simulink model "Aircraft_Power_Network"  (R2015a)
settings: Solver=ode23t  StartTime=0.0  StopTime=40  RelTol=1e-3
PostLoadFcn:
  | %load PQ_DATA4
  | Flight_Cycle_Num = 1;
  | 
  | warning off Simulink:blocks:MatchingFromNotFound
  | warning off Simulink:blocks:MatchingGotoNotFound
  | warning off Simulink:Engine:SaveWithParameterizedLinks_Warning
  | warning off MATLAB:nearlySingularMatrix
  | warning off simscape:compiler:sli:init:SolverNotRecommended
  | warning off Simulink:ID:DuplicateSID
  | warning off Simulink:Engine:UINotUpdatedDuringRapidAccelSim
  | warning off Simulink:SampleTime:IllegalIPortRateTrans
  | warning off Simulink:SampleTime:SourceInheritedTS
StartFcn:
  | tic;
StopFcn:
  | Elapsed_Sim_Time = toc; disp(['Elapsed time is ' num2str(Elapsed_Sim_Time)])
undefined symbols (not defined in the file): sigbuilder_block, Ts
libraries: powerlib x6, powerlib_meascontrol x4, Actuator_AC_Lib x2, Lamp_Lib x2, Pump_Lib x2, DC_Loads_Lib x2, Distribution_Lib x1, Generator_Lib x1, Power_Calc_Lib x1
Description:
  | Copyright 2014 The MathWorks, Inc.
settings Model: CovSFcnEnable=off  TunableVars=Flight_Cycle_Num  TunableVarsStorageClass=Auto  Creator=smiller  LastModifiedBy=dmeissne
settings OptimizationCC: InlineParams=on  OptimizeBlockIOStorage=off  BufferReuse=off  GlobalBufferReuse=off  ExpressionFolding=off  LocalBlockOutputs=off
settings DebuggingCC: UnderspecifiedInitializationDetection=Classic  MergeDetectMultiDrivingBlocksExec=none  SolverPrmCheckMsg=warning  MultiTaskRateTransMsg=warning  StateNameClashWarn=warning
settings GRTTargetCC: CombineOutputUpdateFcns=off  GRTInterface=on

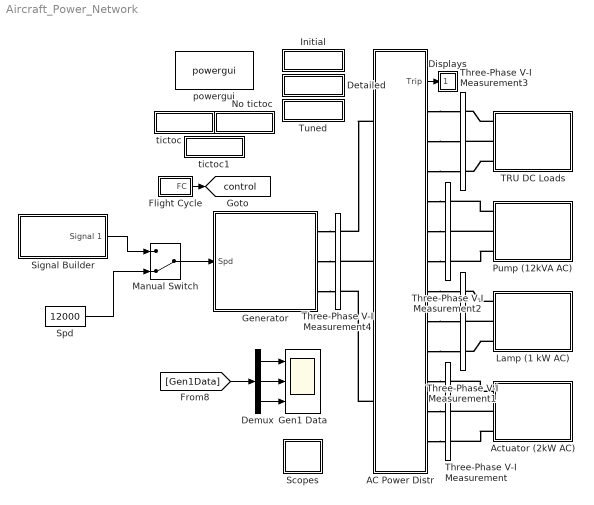
== system Aircraft_Power_Network ==
  AC Power Distr : Subsystem  BlockChoice=Phasor
      settings: AttributesFormatString=%<BlockChoice>  TemplateBlock=Distribution_Lib/AC Power Distr  MemberBlocks=Detailed,Phasor
  Actuator (2kW AC) : Subsystem  BlockChoice=Phasor
      link override Detailed/PM Synchronous Motor Drive/Output Bus Selector: OutputSignals=Rotor speed wm (rad/s)
      link override Detailed/PM Synchronous Motor Drive/Permanent Magnet Synchronous Machine: MechanicalLoad=Torque Tm  VoltageCst=126.966  TorqueCst=1.05
      link override Phasor/Calc PQ: BlockChoice=Tuned
      settings: AttributesFormatString=%<BlockChoice>  TemplateBlock=Actuator_AC_Lib/Actuator (2kW AC)  MemberBlocks=Detailed,Phasor
  Demux : Demux  Outputs=[2 1 1]
  Detailed : Subsystem
      settings: OpenFcn=Select_APN_Model_Config(bdroot,'Detailed');
      mask Display: disp('Detailed');
  Displays : Subsystem
      mask Display: disp('D')
  Flight Cycle : Subsystem
      mask Display: disp(num2str(evalin('base','Flight_Cycle_Num')));
  Gen1 Data : Scope  NumInputPorts=3
      settings: TimeRange=5  YMin=1255~200~5000  YMax=1258~204~20000  SaveName=Gen1_DATA  SampleTime=10e-6
  Generator : Subsystem  BlockChoice=Ideal
      link override VSCF DC Link/DC Link Gen: BlockChoice=Ideal
      link override VSCF DC Link/DC Link Gen/Sync Mach/Simplified Synchronous Machine SI Units/Electrical model: BlockChoice=Phasor
      link override VSCF DC Link/DC Link Gen/Sync Mach/Simplified Synchronous Machine SI Units/From: GotoTag=tp2df5cfb3_b42e_4dd4_aed6_ebb45f5ee09b
      link override VSCF DC Link/DC Link Gen/Sync Mach/Simplified Synchronous Machine SI Units/Goto: GotoTag=tp9f3ab3a0_63ac_4acf_b3bd_c670964be41e
      link override VSCF DC Link/DC Link Gen/Sync Mach/Simplified Synchronous Machine SI Units/Mechanical model: BlockChoice=Phasor w input
      settings: AttributesFormatString=%<BlockChoice>  TemplateBlock=Generator_Lib/Generator  MemberBlocks=Ideal,Integrated Drive,VSCF Cycloconverter,VSCF DC Link
  Initial : Subsystem
      settings: OpenFcn=Select_APN_Model_Config(bdroot,'Initial');
      mask Display: disp('Initial');
  Lamp (1 kW AC) : Subsystem  RequirementInfo={} %GIDa_b4ebd6a2_cdd2_4eca_9ae5_96943b3eee14  BlockChoice=Phasor
      link override Phasor/Calc PQ: BlockChoice=Tuned
      settings: AttributesFormatString=%<BlockChoice>  TemplateBlock=Lamp_Lib/Lamp (1 kW AC)  MemberBlocks=Detailed,Phasor
  Manual Switch : ManualSwitch  CurrentSetting=0
  No tictoc : Subsystem
      settings: OpenFcn=|
      | set_param(bdroot,'StartFcn','');
      | set_param(bdroot,'StopFcn','');
      mask Display: disp('No tictoc')
  Pump (12kVA AC) : Subsystem  BlockChoice=Phasor
      link override Phasor/Calc PQ: BlockChoice=Tuned
      settings: AttributesFormatString=%<BlockChoice>  TemplateBlock=Pump_Lib/Pump (12kVA AC)  MemberBlocks=Detailed,Phasor
  Scopes : Subsystem
  Signal Builder : Subsystem  Tag=STV Subsys  LoadFcn=sigbuilder_block('load');  StartFcn=sigbuilder_block('start');  StopFcn=sigbuilder_block('stop');  ClipboardFcn=sigbuilder_block('clipboard');  mask(Sigbuilder block){}
      mask help: Simulink:masks:SigbuilderBlock_MD
      mask init:
      | if ~strcmp(get_param(bdroot(gcbh),'SimulationStatus'),'stopped') tuvar = sigbuilder_block('maskInit'); end
      settings: CopyFcn=sigbuilder_block('copy');  DeleteFcn=sigbuilder_block('delete');  ModelCloseFcn=sigbuilder_block('modelClose');  PreSaveFcn=sigbuilder_block('preSave');  PauseFcn=sigbuilder_block('pause');  ContinueFcn=sigbuilder_block('continue');  NameChangeFcn=sigbuilder_block('namechange');  OpenFcn=sigbuilder_block('open',[437.6 199.2 550.4 400 ]);  CloseFcn=sigbuilder_block('close');
      mask Display: plot(0, 0, 100, 100,[2, 2, 32, 32, 2], [68, 8, 8, 68, 68],[32, 2], [38, 38], [32, 19, 2],[53, 60, 44], [32, 17, 17, 2],[16, 16, 31, 31]);txt = getActiveGroup(gcbh);text(2, 100, txt,'verticalAlignment', 'top');
  Spd : Constant  Value=12000
  TRU DC Loads : Subsystem  RequirementInfo={'other' 'apn_system_requirements.docx' '@controller_module' 'true' 'TRU Requirements' '' } %GIDa_0f590c74_ec2b_4e2c_b0ce_7c36d608bdaa  BlockChoice=Phasor
      link override Phasor/Calc PQ: BlockChoice=Tuned
      settings: AttributesFormatString=%<BlockChoice>  TemplateBlock=DC_Loads_Lib/TRU DC Loads  MemberBlocks=Detailed,Multidomain,Phasor
  Three-Phase V-I Measurement : powerlib/Measurements/Three-Phase V-I Measurement  VoltageMeasurement=phase-to-ground  SetLabelV=on  LabelV=Vabc_BDMotor  Vpu=off  VpuLL=off  CurrentMeasurement=yes  SetLabelI=on  LabelI=Iabc_BDMotor  Ipu=off  Pbase=100e6  Vbase=500e3  OutputType=Magnitude  PhasorSimulation=on  PSBequivalent=0
  Three-Phase V-I Measurement1 : powerlib/Measurements/Three-Phase V-I Measurement  VoltageMeasurement=phase-to-ground  SetLabelV=on  LabelV=Vabc_Lamp  Vpu=off  VpuLL=off  CurrentMeasurement=yes  SetLabelI=on  LabelI=Iabc_Lamp  Ipu=off  Pbase=100e6  Vbase=500e3  OutputType=Magnitude  PhasorSimulation=on  PSBequivalent=0
  Three-Phase V-I Measurement2 : powerlib/Measurements/Three-Phase V-I Measurement  VoltageMeasurement=phase-to-ground  SetLabelV=on  LabelV=Vabc_InductionMotor  Vpu=off  VpuLL=off  CurrentMeasurement=yes  SetLabelI=on  LabelI=Iabc_InductionMotor  Ipu=off  Pbase=100e6  Vbase=500e3  OutputType=Magnitude  PhasorSimulation=on  PSBequivalent=0
  Three-Phase V-I Measurement3 : powerlib/Measurements/Three-Phase V-I Measurement  VoltageMeasurement=phase-to-ground  SetLabelV=on  LabelV=Vabc_TRU  Vpu=off  VpuLL=off  CurrentMeasurement=yes  SetLabelI=on  LabelI=Iabc_TRU  Ipu=off  Pbase=100e6  Vbase=500e3  OutputType=Magnitude  PhasorSimulation=on  PSBequivalent=0
  Three-Phase V-I Measurement4 : powerlib/Measurements/Three-Phase V-I Measurement  VoltageMeasurement=phase-to-ground  SetLabelV=on  LabelV=Vabc_GEN  Vpu=off  VpuLL=off  CurrentMeasurement=yes  SetLabelI=on  LabelI=Iabc_GEN  Ipu=off  Pbase=100e6  Vbase=500e3  OutputType=Magnitude  PhasorSimulation=on  PSBequivalent=0
  Tuned : Subsystem
      settings: OpenFcn=Select_APN_Model_Config(bdroot,'Tuned');
      mask Display: disp('Tuned');
  powergui : powerlib/powergui  SimulationMode=Phasor  SolverType=Tustin  SampleTime=Ts  frequency=400  SPID=off  DisableSnubberDevices=off  DisableRonSwitches=off  DisableVfSwitches=off  SwTol=0  DisplayEquations=off  Interpol=off  methode=off  Ts=0  FunctionMessages=off  echomessages=off  HookPort=off  EnableUseOfTLC=off  x0status=blocks  frequencyindice=400  Pbase=100e6  ErrMax=0.0001  Iterations=50  UnitsV=kV  UnitsW=MW  buscounter=0  RestoreLinks=no  ResistiveCurrentMeasurement=off  Frange=[0:2:500]  Ylog=off  Xlog=on  ShowGrid=off  save=off  variable=ZData  structure=Gen1_Vab  ZoomFFT=on  StartTime=0.3  cycles=1  DisplayStyle=1  fundamental=400  FreqAxis=on  MaxFrequency=8000  frequencyindicesteady=1  RmsSteady=1  display=off
  tictoc : Subsystem
      settings: OpenFcn=|
      | set_param(bdroot,'StartFcn','tic;');
      | set_param(bdroot,'StopFcn','Elapsed_Sim_Time = toc; disp([''Elapsed time is '' num2str(Elapsed_Sim_Time)])');
      mask Display: disp('tictoc')
  tictoc1 : Subsystem
      settings: OpenFcn=open('APN_Demo_Script.html')
      mask Display: disp('Script')
  tag scope: control=global
  wires:
  Flight Cycle/1(FC) -> [control]
  AC Power Distr/1(Trip) -> Displays/1(In1)
  Spd/1 -> Manual Switch/2
  [Gen1Data] -> Demux/1
  Demux/1 -> Gen1 Data/1
  Demux/2 -> Gen1 Data/2
  Demux/3 -> Gen1 Data/3
  Manual Switch/1 -> Generator/1(Spd)
  Signal Builder/1(Signal 1) -> Manual Switch/1
  connections:
  Generator/RConn1 -- Three-Phase V-I Measurement4/LConn1
  Generator/RConn2 -- Three-Phase V-I Measurement4/LConn2
  Generator/RConn3 -- Three-Phase V-I Measurement4/LConn3
  AC Power Distr/LConn2 -- Three-Phase V-I Measurement4/RConn2
  Lamp (1 kW AC)/LConn3 -- Three-Phase V-I Measurement1/RConn3
  Actuator (2kW AC)/LConn2 -- Three-Phase V-I Measurement/RConn2
  AC Power Distr/RConn3 -- Three-Phase V-I Measurement3/LConn3
  AC Power Distr/RConn6 -- Three-Phase V-I Measurement2/LConn3
  Pump (12kVA AC)/LConn2 -- Three-Phase V-I Measurement2/RConn2
  TRU DC Loads/LConn3 -- Three-Phase V-I Measurement3/RConn3
  Actuator (2kW AC)/LConn3 -- Three-Phase V-I Measurement/RConn3
  Pump (12kVA AC)/LConn3 -- Three-Phase V-I Measurement2/RConn3
  AC Power Distr/RConn4 -- Three-Phase V-I Measurement2/LConn1
  TRU DC Loads/LConn1 -- Three-Phase V-I Measurement3/RConn1
  AC Power Distr/RConn11 -- Three-Phase V-I Measurement/LConn2
  Actuator (2kW AC)/LConn1 -- Three-Phase V-I Measurement/RConn1
  AC Power Distr/RConn8 -- Three-Phase V-I Measurement1/LConn2
  AC Power Distr/LConn3 -- Three-Phase V-I Measurement4/RConn3
  AC Power Distr/LConn1 -- Three-Phase V-I Measurement4/RConn1
  AC Power Distr/RConn12 -- Three-Phase V-I Measurement/LConn3
  AC Power Distr/RConn1 -- Three-Phase V-I Measurement3/LConn1
  AC Power Distr/RConn5 -- Three-Phase V-I Measurement2/LConn2
  AC Power Distr/RConn9 -- Three-Phase V-I Measurement1/LConn3
  TRU DC Loads/LConn2 -- Three-Phase V-I Measurement3/RConn2
  AC Power Distr/RConn7 -- Three-Phase V-I Measurement1/LConn1
  Lamp (1 kW AC)/LConn2 -- Three-Phase V-I Measurement1/RConn2
  AC Power Distr/RConn10 -- Three-Phase V-I Measurement/LConn1
  Lamp (1 kW AC)/LConn1 -- Three-Phase V-I Measurement1/RConn1
  AC Power Distr/RConn2 -- Three-Phase V-I Measurement3/LConn2
  Pump (12kVA AC)/LConn1 -- Three-Phase V-I Measurement2/RConn1

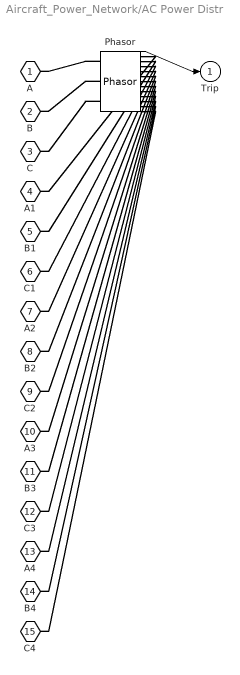
== system Aircraft_Power_Network/AC Power Distr ==
  Phasor : Distribution_Lib/Phasor  FuseA=25  FuseB=200  FuseC=5  FuseD=30
  A : PMIOPort  Port=1  Side=Left
  B : PMIOPort  Port=2  Side=Left
  C : PMIOPort  Port=3  Side=Left
  A1 : PMIOPort  Port=4  Side=Right
  B1 : PMIOPort  Port=5  Side=Right
  C1 : PMIOPort  Port=6  Side=Right
  A2 : PMIOPort  Port=7  Side=Right
  B2 : PMIOPort  Port=8  Side=Right
  C2 : PMIOPort  Port=9  Side=Right
  A3 : PMIOPort  Port=10  Side=Right
  B3 : PMIOPort  Port=11  Side=Right
  C3 : PMIOPort  Port=12  Side=Right
  A4 : PMIOPort  Port=13  Side=Right
  B4 : PMIOPort  Port=14  Side=Right
  C4 : PMIOPort  Port=15  Side=Right
  Trip : Outport
  wires:
  Phasor/1 -> Trip/1
  connections:
  Phasor/LConn1 -- A/RConn1
  Phasor/LConn2 -- B/RConn1
  Phasor/LConn3 -- C/RConn1
  Phasor/RConn1 -- A1/RConn1
  Phasor/RConn2 -- B1/RConn1
  Phasor/RConn3 -- C1/RConn1
  Phasor/RConn4 -- A2/RConn1
  Phasor/RConn5 -- B2/RConn1
  Phasor/RConn6 -- C2/RConn1
  Phasor/RConn7 -- A3/RConn1
  Phasor/RConn8 -- B3/RConn1
  Phasor/RConn9 -- C3/RConn1
  Phasor/RConn10 -- A4/RConn1
  Phasor/RConn11 -- B4/RConn1
  Phasor/RConn12 -- C4/RConn1

== system Aircraft_Power_Network/Actuator (2kW AC) ==
  Phasor : Actuator_AC_Lib/Phasor  SystemSampleTime=-1
  A : PMIOPort  Port=1  Side=Left
  B : PMIOPort  Port=2  Side=Left
  C : PMIOPort  Port=3  Side=Left
  connections:
  Phasor/RConn1 -- A/RConn1
  Phasor/RConn2 -- B/RConn1
  Phasor/RConn3 -- C/RConn1

== system Aircraft_Power_Network/Detailed ==

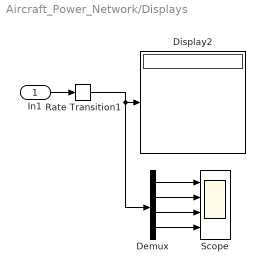
== system Aircraft_Power_Network/Displays ==
  In1 : Inport
  Demux : Demux
  Display2 : Display
      settings: Decimation=100  SampleTime=1e-2
  Rate Transition1 : RateTransition  OutPortSampleTimeOpt=Inherit  OutPortSampleTime=Ts
  Scope : Scope  NumInputPorts=4
      settings: YMin=-5~-5~-5~-5  YMax=5~5~5~5
  wires:
  In1/1 -> Rate Transition1/1
  Rate Transition1/1 -> Demux/1, Display2/1
  Demux/3 -> Scope/3
  Demux/4 -> Scope/4
  Demux/1 -> Scope/1
  Demux/2 -> Scope/2

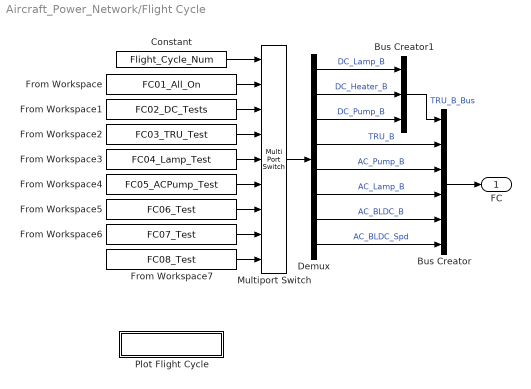
== system Aircraft_Power_Network/Flight Cycle ==
  Bus Creator : BusCreator  Inputs=6
  Bus Creator1 : BusCreator  Inputs=3
  Constant : Constant  Value=Flight_Cycle_Num
  Demux : Demux  Outputs=8
  From Workspace : FromWorkspace  VariableName=FC01_All_On  SampleTime=0  OutputAfterFinalValue=Holding final value
  From Workspace1 : FromWorkspace  VariableName=FC02_DC_Tests  SampleTime=0
  From Workspace2 : FromWorkspace  VariableName=FC03_TRU_Test  SampleTime=0
  From Workspace3 : FromWorkspace  VariableName=FC04_Lamp_Test  SampleTime=0
  From Workspace4 : FromWorkspace  VariableName=FC05_ACPump_Test  SampleTime=0  OutputAfterFinalValue=Holding final value
  From Workspace5 : FromWorkspace  VariableName=FC06_Test  SampleTime=0  OutputAfterFinalValue=Holding final value
  From Workspace6 : FromWorkspace  VariableName=FC07_Test  SampleTime=0  OutputAfterFinalValue=Holding final value
  From Workspace7 : FromWorkspace  VariableName=FC08_Test  SampleTime=0  OutputAfterFinalValue=Holding final value
  Multiport Switch : MultiPortSwitch  Inputs=8
  Plot Flight Cycle : Subsystem
      settings: OpenFcn=Plot_FC
      mask Display: disp('Plot Flight Cycle');
  FC : Outport
  wires:
  Bus Creator/1 -> FC/1
  Bus Creator1/1 -> Bus Creator/1  "TRU_B_Bus"
  From Workspace/1 -> Multiport Switch/2
  From Workspace1/1 -> Multiport Switch/3
  From Workspace2/1 -> Multiport Switch/4
  From Workspace3/1 -> Multiport Switch/5
  From Workspace4/1 -> Multiport Switch/6
  Multiport Switch/1 -> Demux/1
  Constant/1 -> Multiport Switch/1
  Demux/1 -> Bus Creator1/1  "DC_Lamp_B"
  Demux/2 -> Bus Creator1/2  "DC_Heater_B"
  Demux/3 -> Bus Creator1/3  "DC_Pump_B"
  Demux/4 -> Bus Creator/2  "TRU_B"
  Demux/5 -> Bus Creator/3  "AC_Pump_B"
  Demux/6 -> Bus Creator/4  "AC_Lamp_B"
  Demux/7 -> Bus Creator/5  "AC_BLDC_B"
  Demux/8 -> Bus Creator/6  "AC_BLDC_Spd"
  From Workspace5/1 -> Multiport Switch/7
  From Workspace6/1 -> Multiport Switch/8
  From Workspace7/1 -> Multiport Switch/9

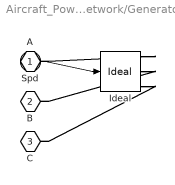
== system Aircraft_Power_Network/Generator ==
  Spd : Inport
  Ideal : Generator_Lib/Ideal  SystemSampleTime=-1
  A : PMIOPort  Port=1  Side=Right
  B : PMIOPort  Port=2  Side=Right
  C : PMIOPort  Port=3  Side=Right
  wires:
  Spd/1 -> Ideal/1
  connections:
  Ideal/RConn1 -- A/RConn1
  Ideal/RConn2 -- B/RConn1
  Ideal/RConn3 -- C/RConn1

== system Aircraft_Power_Network/Initial ==

== system Aircraft_Power_Network/Lamp (1 kW AC) ==
  Phasor : Lamp_Lib/Phasor  SystemSampleTime=-1
  A : PMIOPort  Port=1  Side=Left
  B : PMIOPort  Port=2  Side=Left
  C : PMIOPort  Port=3  Side=Left
  connections:
  Phasor/LConn1 -- A/RConn1
  Phasor/LConn2 -- B/RConn1
  Phasor/LConn3 -- C/RConn1

== system Aircraft_Power_Network/No tictoc ==

== system Aircraft_Power_Network/Pump (12kVA AC) ==
  Phasor : Pump_Lib/Phasor  SystemSampleTime=-1
  A : PMIOPort  Port=1  Side=Left
  B : PMIOPort  Port=2  Side=Left
  C : PMIOPort  Port=3  Side=Left
  connections:
  Phasor/LConn1 -- A/RConn1
  Phasor/LConn2 -- B/RConn1
  Phasor/LConn3 -- C/RConn1

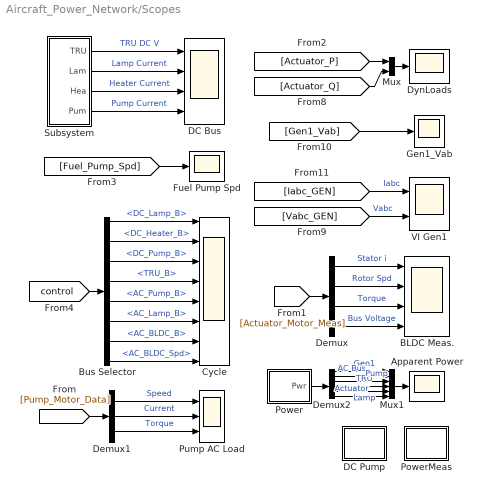
== system Aircraft_Power_Network/Scopes ==
  Apparent Power : Scope
      settings: ShowLegends=on  YMin=-25000  YMax=45000  SaveName=data  Decimation=10  SampleTime=10e-6
  BLDC Meas. : Scope  NumInputPorts=4
      settings: YMin=-20~-600~-30~250  YMax=20~600~30~300  SaveName=simout  Decimation=10
  Bus Selector : BusSelector  OutputSignals=TRU_B_Bus.DC_Lamp_B,TRU_B_Bus.DC_Heater_B,TRU_B_Bus.DC_Pump_B,TRU_B,AC_Pump_B,AC_Lamp_B,AC_BLDC_B,AC_BLDC_Spd
  Cycle : Scope  NumInputPorts=8
      settings: YMin=-5~-5~-5~-5~-5~-5~-5~-5  YMax=5~5~5~5~5~5~5~5  SaveName=ScopeData3
  DC Bus : Scope  NumInputPorts=4
      settings: YMin=-10~-10~-10~-5  YMax=50~50~100~5  SaveName=vac  Decimation=10  SampleTime=10e-6
  DC Pump : Subsystem
  Demux : Demux  Outputs=[1 2 2 1]
  Demux1 : Demux  Outputs=3
  Demux2 : Demux  Outputs=6
  DynLoads : Scope
      settings: TimeRange=5  YMin=-100  YMax=1000  SaveName=vac1  SampleTime=10e-6
  Fuel Pump Spd : Scope
      settings: TimeRange=5  YMin=0  YMax=250  SaveName=data1  Decimation=10  SampleTime=10e-6
  Gen1_Vab : Scope
      settings: TimeRange=0.005  YMin=-400  YMax=400  SaveName=Gen1_Vab
  Mux : Mux  Inputs=2
  Mux1 : Mux  Inputs=6
  Power : Subsystem
  PowerMeas : Subsystem
  Pump AC Load : Scope  NumInputPorts=3
      settings: TimeRange=5  YMin=295~-100~-40  YMax=315~200~40  SaveName=IM  Decimation=100  SampleTime=1e-3
  Subsystem : Subsystem
  VI Gen1 : Scope  NumInputPorts=2
      settings: TimeRange=5  YMin=-200~-200  YMax=200~200  SaveName=IabcGEN  SampleTime=10e-6
  wires:
  [Fuel_Pump_Spd] -> Fuel Pump Spd/1
  Demux/1 -> BLDC Meas./1  "Stator i"
  Demux/2 -> BLDC Meas./2  "Rotor Spd"
  Demux/3 -> BLDC Meas./3  "Torque"
  Demux/4 -> BLDC Meas./4  "Bus Voltage"
  [Actuator_Motor_Meas] -> Demux/1
  Subsystem/2(Lam) -> DC Bus/2  "Lamp Current"
  Subsystem/3(Hea) -> DC Bus/3  "Heater Current"
  Subsystem/4(Pum) -> DC Bus/4  "Pump Current"
  Subsystem/1(TRU) -> DC Bus/1  "TRU DC V"
  [Gen1_Vab] -> Gen1_Vab/1
  [control] -> Bus Selector/1
  Bus Selector/8 -> Cycle/8  "<AC_BLDC_Spd>"
  Bus Selector/7 -> Cycle/7  "<AC_BLDC_B>"
  Bus Selector/5 -> Cycle/5  "<AC_Pump_B>"
  Bus Selector/6 -> Cycle/6  "<AC_Lamp_B>"
  Bus Selector/1 -> Cycle/1  "<DC_Lamp_B>"
  Bus Selector/2 -> Cycle/2  "<DC_Heater_B>"
  Bus Selector/4 -> Cycle/4  "<TRU_B>"
  Bus Selector/3 -> Cycle/3  "<DC_Pump_B>"
  [Actuator_P] -> Mux/1
  Mux/1 -> DynLoads/1
  [Actuator_Q] -> Mux/2
  [Iabc_GEN] -> VI Gen1/1  "Iabc"
  [Vabc_GEN] -> VI Gen1/2  "Vabc"
  Power/1(Pwr) -> Demux2/1
  Demux1/3 -> Pump AC Load/3  "Torque"
  Demux1/1 -> Pump AC Load/1  "Speed"
  Demux1/2 -> Pump AC Load/2  "Current"
  [Pump_Motor_Data] -> Demux1/1
  Demux2/6 -> Mux1/6  "Actuator"
  Demux2/1 -> Mux1/1  "Gen1"
  Demux2/2 -> Mux1/2  "AC Bus"
  Demux2/4 -> Mux1/4  "TRU"
  Demux2/3 -> Mux1/3  "Pump"
  Demux2/5 -> Mux1/5  "Lamp"
  Mux1/1 -> Apparent Power/1

== system Aircraft_Power_Network/Signal Builder ==
  Demux : Demux  Tag=STV Demux  Outputs=1
  FromWs : FromWorkspace  Tag=STV FromWs  VariableName=tuvar  SampleTime=0
      SigBuilderData=|
      | common.afterFinalStr = 'Extrapolate'
      | common.sampleTime = 0
      | dataSet.timeRange = [0 10]
      | dataSet.name = 'Group 1'
      | sbobj.Groups.Name = 'Group 1'
      | sbobj.Groups.Signals.Name = 'Signal 1'
      | sbobj.Groups.Signals.XData = [0 10]
      | sbobj.Groups.Signals.YData = [1 1.005]
  Signal 1 : Outport  Tag=STV Outport
  wires:
  Demux/1 -> Signal 1/1
  FromWs/1 -> Demux/1

== system Aircraft_Power_Network/TRU DC Loads ==
  Phasor : DC_Loads_Lib/Phasor  SystemSampleTime=-1
  A : PMIOPort  Port=1  Side=Left
  B : PMIOPort  Port=2  Side=Left
  C : PMIOPort  Port=3  Side=Left
  connections:
  Phasor/LConn1 -- A/RConn1
  Phasor/LConn2 -- B/RConn1
  Phasor/LConn3 -- C/RConn1

== system Aircraft_Power_Network/Tuned ==

== system Aircraft_Power_Network/tictoc ==

== system Aircraft_Power_Network/tictoc1 ==

== system Aircraft_Power_Network/Flight Cycle/Plot Flight Cycle ==

== system Aircraft_Power_Network/Scopes/DC Pump ==
  DC Bus1 : Scope  NumInputPorts=3
      settings: YMin=-10~-10~-10  YMax=50~50~100  SaveName=vac2  Decimation=10  SampleTime=10e-6
  wires:
  [PumpDC_i] -> DC Bus1/2
  [PumpDC_Spd] -> DC Bus1/1
  [PumpDC_Trq] -> DC Bus1/3

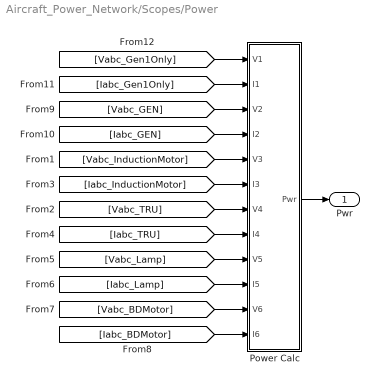
== system Aircraft_Power_Network/Scopes/Power ==
  Power Calc : Subsystem  BlockChoice=Phasor
      settings: AttributesFormatString=%<BlockChoice>  TemplateBlock=Power_Calc_Lib/Power Calc  MemberBlocks=Detailed,Phasor
  Pwr : Outport
  wires:
  [Vabc_Gen1Only] -> Power Calc/1(V1)
  [Iabc_Gen1Only] -> Power Calc/2(I1)
  [Vabc_GEN] -> Power Calc/3(V2)
  [Iabc_GEN] -> Power Calc/4(I2)
  [Vabc_InductionMotor] -> Power Calc/5(V3)
  [Iabc_InductionMotor] -> Power Calc/6(I3)
  [Vabc_TRU] -> Power Calc/7(V4)
  [Iabc_TRU] -> Power Calc/8(I4)
  [Vabc_Lamp] -> Power Calc/9(V5)
  [Iabc_Lamp] -> Power Calc/10(I5)
  Power Calc/1(Pwr) -> Pwr/1
  [Vabc_BDMotor] -> Power Calc/11(V6)
  [Iabc_BDMotor] -> Power Calc/12(I6)

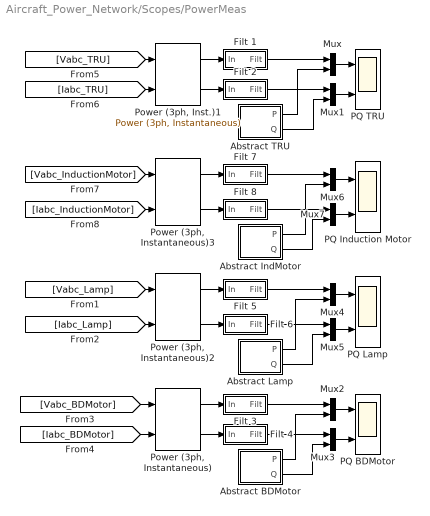
== system Aircraft_Power_Network/Scopes/PowerMeas ==
  Abstract BDMotor : Subsystem
  Abstract IndMotor : Subsystem
  Abstract Lamp : Subsystem
  Abstract TRU : Subsystem
  Filt 1 : Subsystem
  Filt 2 : Subsystem
  Filt 3 : Subsystem
  Filt 4 : Subsystem
  Filt 5 : Subsystem
  Filt 6 : Subsystem
  Filt 7 : Subsystem
  Filt 8 : Subsystem
  Mux{,1..7} (8 alike) : Mux  Inputs=2
  PQ BDMotor : Scope  NumInputPorts=2
      settings: TimeRange=5  YMin=-200~-200  YMax=1400~800  SaveName=PQ_BDMotor  Decimation=100  SampleTime=10e-6
  PQ Induction Motor : Scope  NumInputPorts=2
      settings: TimeRange=5  YMin=0~-1000  YMax=10000~0  SaveName=PQ_InductionMotor  Decimation=100  SampleTime=10e-6
  PQ Lamp : Scope  NumInputPorts=2
      settings: TimeRange=5  YMin=-500~-200  YMax=1500~800  SaveName=PQ_Lamp  Decimation=100  SampleTime=10e-6
  PQ TRU : Scope  NumInputPorts=2
      settings: YMin=0~-1000  YMax=6000~1000  SaveName=PQ_TRU  Decimation=100  SampleTime=10e-6
  "Power (3ph, Instantaneous)" : powerlib_meascontrol/Measurements/Power (3ph, Instantaneous)
  "Power (3ph, Instantaneous)2" : powerlib_meascontrol/Measurements/Power (3ph, Instantaneous)
  "Power (3ph, Instantaneous)3" : powerlib_meascontrol/Measurements/Power (3ph, Instantaneous)
  "Power (3ph, Inst.)1" : powerlib_meascontrol/Measurements/Power (3ph, Instantaneous)
  wires:
  Filt 3/1(Filt) -> Mux2/1
  [Vabc_BDMotor] -> "Power (3ph, Instantaneous)"/1
  [Iabc_TRU] -> "Power (3ph, Inst.)1"/2
  Filt 1/1(Filt) -> Mux/1
  "Power (3ph, Inst.)1"/2 -> Filt 2/1(In)
  "Power (3ph, Instantaneous)"/1 -> Filt 3/1(In)
  [Iabc_BDMotor] -> "Power (3ph, Instantaneous)"/2
  "Power (3ph, Instantaneous)"/2 -> Filt 4/1(In)
  Filt 2/1(Filt) -> Mux1/1
  [Vabc_TRU] -> "Power (3ph, Inst.)1"/1
  "Power (3ph, Inst.)1"/1 -> Filt 1/1(In)
  Filt 4/1(Filt) -> Mux3/1
  [Iabc_Lamp] -> "Power (3ph, Instantaneous)2"/2
  "Power (3ph, Instantaneous)2"/2 -> Filt 6/1(In)
  [Vabc_Lamp] -> "Power (3ph, Instantaneous)2"/1
  "Power (3ph, Instantaneous)2"/1 -> Filt 5/1(In)
  [Iabc_InductionMotor] -> "Power (3ph, Instantaneous)3"/2
  Filt 7/1(Filt) -> Mux6/1
  "Power (3ph, Instantaneous)3"/2 -> Filt 8/1(In)
  Filt 8/1(Filt) -> Mux7/1
  [Vabc_InductionMotor] -> "Power (3ph, Instantaneous)3"/1
  "Power (3ph, Instantaneous)3"/1 -> Filt 7/1(In)
  Mux/1 -> PQ TRU/1
  Mux1/1 -> PQ TRU/2
  Mux2/1 -> PQ BDMotor/1
  Mux3/1 -> PQ BDMotor/2
  Filt 5/1(Filt) -> Mux4/1
  Filt 6/1(Filt) -> Mux5/1
  Mux4/1 -> PQ Lamp/1
  Mux5/1 -> PQ Lamp/2
  Abstract TRU/1(P) -> Mux/2
  Abstract TRU/2(Q) -> Mux1/2
  Abstract BDMotor/1(P) -> Mux2/2
  Abstract BDMotor/2(Q) -> Mux3/2
  Abstract Lamp/1(P) -> Mux4/2
  Abstract Lamp/2(Q) -> Mux5/2
  Mux6/1 -> PQ Induction Motor/1
  Mux7/1 -> PQ Induction Motor/2
  Abstract IndMotor/1(P) -> Mux6/2
  Abstract IndMotor/2(Q) -> Mux7/2

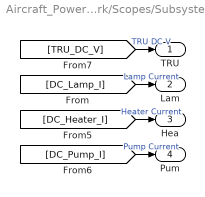
== system Aircraft_Power_Network/Scopes/Subsystem ==
  TRU : Outport
  Lam : Outport  Port=2
  Hea : Outport  Port=3
  Pum : Outport  Port=4
  wires:
  [DC_Lamp_I] -> Lam/1  "Lamp Current"
  [DC_Pump_I] -> Pum/1  "Pump Current"
  [DC_Heater_I] -> Hea/1  "Heater Current"
  [TRU_DC_V] -> TRU/1  "TRU DC V"

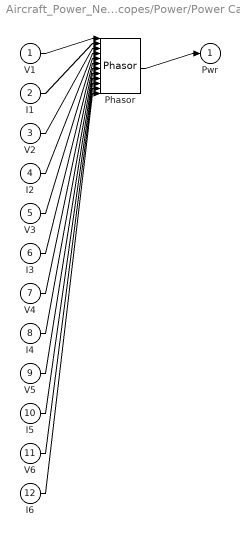
== system Aircraft_Power_Network/Scopes/Power/Power Calc ==
  V1 : Inport
  I1 : Inport  Port=2
  V2 : Inport  Port=3
  I2 : Inport  Port=4
  V3 : Inport  Port=5
  I3 : Inport  Port=6
  V4 : Inport  Port=7
  I4 : Inport  Port=8
  V5 : Inport  Port=9
  I5 : Inport  Port=10
  V6 : Inport  Port=11
  I6 : Inport  Port=12
  Phasor : Power_Calc_Lib/Phasor
  Pwr : Outport
  wires:
  V1/1 -> Phasor/1
  I1/1 -> Phasor/2
  V2/1 -> Phasor/3
  I2/1 -> Phasor/4
  V3/1 -> Phasor/5
  I3/1 -> Phasor/6
  V4/1 -> Phasor/7
  I4/1 -> Phasor/8
  V5/1 -> Phasor/9
  I5/1 -> Phasor/10
  V6/1 -> Phasor/11
  I6/1 -> Phasor/12
  Phasor/1 -> Pwr/1

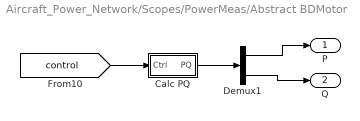
== system Aircraft_Power_Network/Scopes/PowerMeas/Abstract BDMotor ==
  Calc PQ : Subsystem  BlockChoice=Tuned
      settings: AttributesFormatString=%<BlockChoice>  TemplateBlock=Actuator_AC_Lib/Calc PQ  MemberBlocks=Initial,Tuned
  Demux1 : Demux  Outputs=2
  P : Outport
  Q : Outport  Port=2
  wires:
  [control] -> Calc PQ/1(Ctrl)
  Calc PQ/1(PQ) -> Demux1/1
  Demux1/1 -> P/1
  Demux1/2 -> Q/1

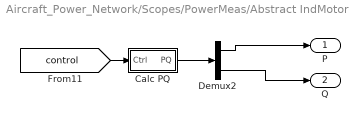
== system Aircraft_Power_Network/Scopes/PowerMeas/Abstract IndMotor ==
  Calc PQ : Subsystem  BlockChoice=Tuned
      settings: AttributesFormatString=%<BlockChoice>  TemplateBlock=Pump_Lib/Calc PQ  MemberBlocks=Initial,Tuned
  Demux2 : Demux  Outputs=2
  P : Outport
  Q : Outport  Port=2
  wires:
  Calc PQ/1(PQ) -> Demux2/1
  Demux2/2 -> Q/1
  Demux2/1 -> P/1
  [control] -> Calc PQ/1(Ctrl)

== system Aircraft_Power_Network/Scopes/PowerMeas/Abstract Lamp ==
  Calc PQ : Subsystem  BlockChoice=Tuned
      settings: AttributesFormatString=%<BlockChoice>  TemplateBlock=Lamp_Lib/Calc PQ  MemberBlocks=Initial,Tuned
  Demux2 : Demux  Outputs=2
  P : Outport
  Q : Outport  Port=2
  wires:
  [control] -> Calc PQ/1(Ctrl)
  Demux2/1 -> P/1
  Demux2/2 -> Q/1
  Calc PQ/1(PQ) -> Demux2/1

== system Aircraft_Power_Network/Scopes/PowerMeas/Abstract TRU ==
  Calc PQ : Subsystem  BlockChoice=Tuned
      settings: AttributesFormatString=%<BlockChoice>  TemplateBlock=DC_Loads_Lib/Calc PQ  MemberBlocks=Initial,Tuned
  Demux : Demux  Outputs=2
  P : Outport
  Q : Outport  Port=2
  wires:
  [control] -> Calc PQ/1(Ctrl)
  Calc PQ/1(PQ) -> Demux/1
  Demux/1 -> P/1
  Demux/2 -> Q/1

== system Aircraft_Power_Network/Scopes/PowerMeas/Filt 1 ==
  In : Inport
  Mux : Mux  Inputs=2
  Transfer Fcn : TransferFcn  Denominator=[0.01 1]
  Filt : Outport
  wires:
  Transfer Fcn/1 -> Mux/2
  In/1 -> Transfer Fcn/1, Mux/1
  Mux/1 -> Filt/1

== system Aircraft_Power_Network/Scopes/PowerMeas/Filt 2 ==
  In : Inport
  Mux : Mux  Inputs=2
  Transfer Fcn : TransferFcn  Denominator=[0.01 1]
  Filt : Outport
  wires:
  Mux/1 -> Filt/1
  In/1 -> Mux/1, Transfer Fcn/1
  Transfer Fcn/1 -> Mux/2

== system Aircraft_Power_Network/Scopes/PowerMeas/Filt 3 ==
  In : Inport
  Mux : Mux  Inputs=2
  Transfer Fcn : TransferFcn  Denominator=[0.01 1]
  Filt : Outport
  wires:
  Transfer Fcn/1 -> Mux/2
  In/1 -> Transfer Fcn/1, Mux/1
  Mux/1 -> Filt/1

== system Aircraft_Power_Network/Scopes/PowerMeas/Filt 4 ==
  In : Inport
  Mux : Mux  Inputs=2
  Transfer Fcn : TransferFcn  Denominator=[0.01 1]
  Filt : Outport
  wires:
  Mux/1 -> Filt/1
  In/1 -> Mux/1, Transfer Fcn/1
  Transfer Fcn/1 -> Mux/2

== system Aircraft_Power_Network/Scopes/PowerMeas/Filt 5 ==
  In : Inport
  Mux : Mux  Inputs=2
  Transfer Fcn : TransferFcn  Denominator=[0.01 1]
  Filt : Outport
  wires:
  Transfer Fcn/1 -> Mux/2
  In/1 -> Transfer Fcn/1, Mux/1
  Mux/1 -> Filt/1

== system Aircraft_Power_Network/Scopes/PowerMeas/Filt 6 ==
  In : Inport
  Mux : Mux  Inputs=2
  Transfer Fcn : TransferFcn  Denominator=[0.01 1]
  Filt : Outport
  wires:
  Mux/1 -> Filt/1
  In/1 -> Mux/1, Transfer Fcn/1
  Transfer Fcn/1 -> Mux/2

== system Aircraft_Power_Network/Scopes/PowerMeas/Filt 7 ==
  In : Inport
  Mux : Mux  Inputs=2
  Transfer Fcn : TransferFcn  Denominator=[0.01 1]
  Filt : Outport
  wires:
  Transfer Fcn/1 -> Mux/2
  In/1 -> Transfer Fcn/1, Mux/1
  Mux/1 -> Filt/1

== system Aircraft_Power_Network/Scopes/PowerMeas/Filt 8 ==
  In : Inport
  Mux : Mux  Inputs=2
  Transfer Fcn : TransferFcn  Denominator=[0.01 1]
  Filt : Outport
  wires:
  Mux/1 -> Filt/1
  In/1 -> Mux/1, Transfer Fcn/1
  Transfer Fcn/1 -> Mux/2

== system Aircraft_Power_Network/Scopes/PowerMeas/Abstract BDMotor/Calc PQ ==
  Ctrl : Inport
  Tuned : Actuator_AC_Lib/Tuned
  PQ : Outport
  wires:
  Ctrl/1 -> Tuned/1
  Tuned/1 -> PQ/1

== system Aircraft_Power_Network/Scopes/PowerMeas/Abstract IndMotor/Calc PQ ==
  Ctrl : Inport
  Tuned : Pump_Lib/Tuned
  PQ : Outport
  wires:
  Ctrl/1 -> Tuned/1
  Tuned/1 -> PQ/1

== system Aircraft_Power_Network/Scopes/PowerMeas/Abstract Lamp/Calc PQ ==
  Ctrl : Inport
  Tuned : Lamp_Lib/Tuned
  PQ : Outport
  wires:
  Ctrl/1 -> Tuned/1
  Tuned/1 -> PQ/1

== system Aircraft_Power_Network/Scopes/PowerMeas/Abstract TRU/Calc PQ ==
  Ctrl : Inport
  Tuned : DC_Loads_Lib/Tuned
  PQ : Outport
  wires:
  Ctrl/1 -> Tuned/1
  Tuned/1 -> PQ/1
